simulink model "PID_controler"  (R2022b)
settings: Solver=FixedStepAuto  StartTime=0.0  StopTime=10.0  FixedStep=1e-3  MaxStep=1e-3  RelTol=1e-3
(part 1 of 2)
settings Model: Creator=MAAM  LastModifiedBy=MAAM

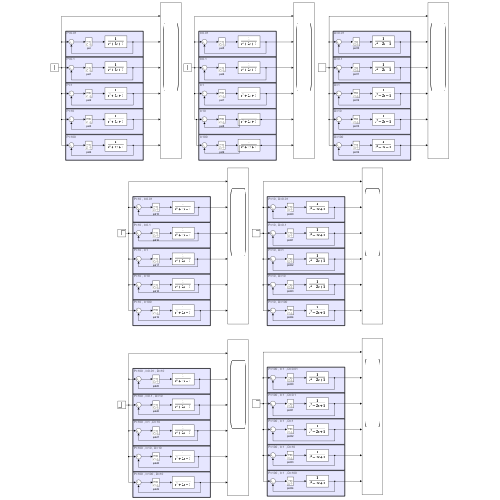
[thumbnail: Simulink's stored preview of the top-level diagram]
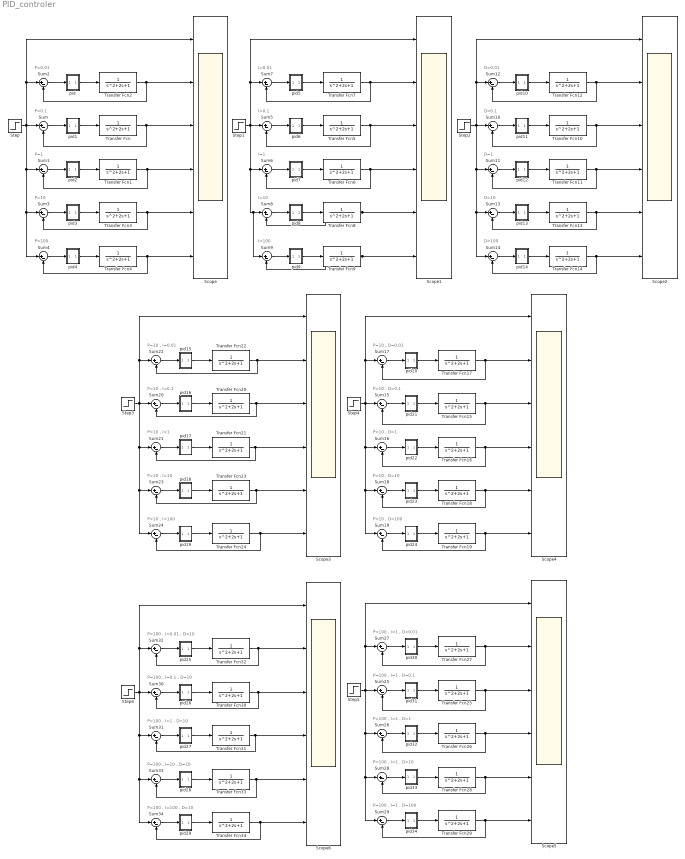
== system PID_controler ==
  note: P=0.1
  note: P=1
  note: P=0.01
  note: P=10
  note: P=100
  note: I=0.1
  note: I=1
  note: I=0.01
  note: I=10
  note: I=100
  note: D=0.1
  note: D=1
  note: D=0.01
  note: D=10
  note: D=100
  note: P=10 , I=0.1
  note: P=10 , I=1
  note: P=10 , I=0.01
  note: P=10 , I=10
  note: P=10 , I=100
  note: P=10 , D=0.1
  note: P=10 , D=1
  note: P=10 , D=0.01
  note: P=10 , D=10
  note: P=10 , D=100
  note: P=100 , I=1 , D=0.1
  note: P=100 , I=1 , D=1
  note: P=100 , I=1 , D=0.01
  note: P=100 , I=1 , D=10
  note: P=100 , I=1 , D=100
  note: P=100 , I=0.1 , D=10
  note: P=100 , I=1 , D=10
  note: P=100 , I=0.01 , D=10
  note: P=100 , I=10 , D=10
  note: P=100 , I=100 , D=10
  Scope{,1..6} (7 alike) : Scope  NumInputPorts=6
  Step{,1..6} (7 alike) : Step  SampleTime=0
  Sum{,1..34} (35 alike) : Sum  Inputs=|+-
  Transfer Fcn{,1..34} (35 alike) : TransferFcn
  pid : Subsystem  Variant=on  mask{F=Parallel, P=0.01, I=0, D=0}
      mask prompts: F "Form"; P "Propotional (P):"; I "Integral      (I):"; D "Drivative    (D):"
      mask init:
      | % Ensure parameters are initialized correctly
      | if isempty(P)
      |     P = 0;
      | end
      | if isempty(I)
      |     I = 0;
      | end
      | if isempty(D)
      |     D = 0;
      | end
      mask TypeOptions F: Parallel | Series | Ideal
      mask TypeOptions P: Subsystem/Gain/Gain | Subsystem1/Gain/Gain | Subsystem2/Gain/Gain
      mask TypeOptions I: Subsystem/Gain1/Gain | Subsystem1/Gain1/Gain | Subsystem2/Gain1/Gain
      mask TypeOptions D: Subsystem/Gain2/Gain | Subsystem1/Gain2/Gain | Subsystem2/Gain2/Gain
      mask Display: fprintf('PID');
  pid1 : Subsystem  Variant=on  mask{F=Parallel, P=0.1, I=0, D=0}
      mask prompts: F "Form"; P "Propotional (P):"; I "Integral      (I):"; D "Drivative    (D):"
      mask init:
      | % Ensure parameters are initialized correctly
      | if isempty(P)
      |     P = 0;
      | end
      | if isempty(I)
      |     I = 0;
      | end
      | if isempty(D)
      |     D = 0;
      | end
      mask TypeOptions F: Parallel | Series | Ideal
      mask TypeOptions P: Subsystem/Gain/Gain | Subsystem1/Gain/Gain | Subsystem2/Gain/Gain
      mask TypeOptions I: Subsystem/Gain1/Gain | Subsystem1/Gain1/Gain | Subsystem2/Gain1/Gain
      mask TypeOptions D: Subsystem/Gain2/Gain | Subsystem1/Gain2/Gain | Subsystem2/Gain2/Gain
      mask Display: fprintf('PID');
  pid10 : Subsystem  Variant=on  mask{F=Parallel, P=0, I=0, D=0.01}
      mask prompts: F "Form"; P "Propotional (P):"; I "Integral      (I):"; D "Drivative    (D):"
      mask init:
      | % Ensure parameters are initialized correctly
      | if isempty(P)
      |     P = 0;
      | end
      | if isempty(I)
      |     I = 0;
      | end
      | if isempty(D)
      |     D = 0;
      | end
      mask TypeOptions F: Parallel | Series | Ideal
      mask TypeOptions P: Subsystem/Gain/Gain | Subsystem1/Gain/Gain | Subsystem2/Gain/Gain
      mask TypeOptions I: Subsystem/Gain1/Gain | Subsystem1/Gain1/Gain | Subsystem2/Gain1/Gain
      mask TypeOptions D: Subsystem/Gain2/Gain | Subsystem1/Gain2/Gain | Subsystem2/Gain2/Gain
      mask Display: fprintf('PID');
  pid11 : Subsystem  Variant=on  mask{F=Parallel, P=0, I=0, D=0.1}
      mask prompts: F "Form"; P "Propotional (P):"; I "Integral      (I):"; D "Drivative    (D):"
      mask init:
      | % Ensure parameters are initialized correctly
      | if isempty(P)
      |     P = 0;
      | end
      | if isempty(I)
      |     I = 0;
      | end
      | if isempty(D)
      |     D = 0;
      | end
      mask TypeOptions F: Parallel | Series | Ideal
      mask TypeOptions P: Subsystem/Gain/Gain | Subsystem1/Gain/Gain | Subsystem2/Gain/Gain
      mask TypeOptions I: Subsystem/Gain1/Gain | Subsystem1/Gain1/Gain | Subsystem2/Gain1/Gain
      mask TypeOptions D: Subsystem/Gain2/Gain | Subsystem1/Gain2/Gain | Subsystem2/Gain2/Gain
      mask Display: fprintf('PID');
  pid12 : Subsystem  Variant=on  mask{F=Parallel, P=0, I=0, D=1}
      mask prompts: F "Form"; P "Propotional (P):"; I "Integral      (I):"; D "Drivative    (D):"
      mask init:
      | % Ensure parameters are initialized correctly
      | if isempty(P)
      |     P = 0;
      | end
      | if isempty(I)
      |     I = 0;
      | end
      | if isempty(D)
      |     D = 0;
      | end
      mask TypeOptions F: Parallel | Series | Ideal
      mask TypeOptions P: Subsystem/Gain/Gain | Subsystem1/Gain/Gain | Subsystem2/Gain/Gain
      mask TypeOptions I: Subsystem/Gain1/Gain | Subsystem1/Gain1/Gain | Subsystem2/Gain1/Gain
      mask TypeOptions D: Subsystem/Gain2/Gain | Subsystem1/Gain2/Gain | Subsystem2/Gain2/Gain
      mask Display: fprintf('PID');
  pid13 : Subsystem  Variant=on  mask{F=Parallel, P=0, I=0, D=10}
      mask prompts: F "Form"; P "Propotional (P):"; I "Integral      (I):"; D "Drivative    (D):"
      mask init:
      | % Ensure parameters are initialized correctly
      | if isempty(P)
      |     P = 0;
      | end
      | if isempty(I)
      |     I = 0;
      | end
      | if isempty(D)
      |     D = 0;
      | end
      mask TypeOptions F: Parallel | Series | Ideal
      mask TypeOptions P: Subsystem/Gain/Gain | Subsystem1/Gain/Gain | Subsystem2/Gain/Gain
      mask TypeOptions I: Subsystem/Gain1/Gain | Subsystem1/Gain1/Gain | Subsystem2/Gain1/Gain
      mask TypeOptions D: Subsystem/Gain2/Gain | Subsystem1/Gain2/Gain | Subsystem2/Gain2/Gain
      mask Display: fprintf('PID');
  pid14 : Subsystem  Variant=on  mask{F=Parallel, P=0, I=0, D=100}
      mask prompts: F "Form"; P "Propotional (P):"; I "Integral      (I):"; D "Drivative    (D):"
      mask init:
      | % Ensure parameters are initialized correctly
      | if isempty(P)
      |     P = 0;
      | end
      | if isempty(I)
      |     I = 0;
      | end
      | if isempty(D)
      |     D = 0;
      | end
      mask TypeOptions F: Parallel | Series | Ideal
      mask TypeOptions P: Subsystem/Gain/Gain | Subsystem1/Gain/Gain | Subsystem2/Gain/Gain
      mask TypeOptions I: Subsystem/Gain1/Gain | Subsystem1/Gain1/Gain | Subsystem2/Gain1/Gain
      mask TypeOptions D: Subsystem/Gain2/Gain | Subsystem1/Gain2/Gain | Subsystem2/Gain2/Gain
      mask Display: fprintf('PID');
  pid15 : Subsystem  Variant=on  mask{F=Parallel, P=100, I=0.01, D=0}
      mask prompts: F "Form"; P "Propotional (P):"; I "Integral      (I):"; D "Drivative    (D):"
      mask init:
      | % Ensure parameters are initialized correctly
      | if isempty(P)
      |     P = 0;
      | end
      | if isempty(I)
      |     I = 0;
      | end
      | if isempty(D)
      |     D = 0;
      | end
      mask TypeOptions F: Parallel | Series | Ideal
      mask TypeOptions P: Subsystem/Gain/Gain | Subsystem1/Gain/Gain | Subsystem2/Gain/Gain
      mask TypeOptions I: Subsystem/Gain1/Gain | Subsystem1/Gain1/Gain | Subsystem2/Gain1/Gain
      mask TypeOptions D: Subsystem/Gain2/Gain | Subsystem1/Gain2/Gain | Subsystem2/Gain2/Gain
      mask Display: fprintf('PID');
  pid16 : Subsystem  Variant=on  mask{F=Parallel, P=100, I=0.1, D=0}
      mask prompts: F "Form"; P "Propotional (P):"; I "Integral      (I):"; D "Drivative    (D):"
      mask init:
      | % Ensure parameters are initialized correctly
      | if isempty(P)
      |     P = 0;
      | end
      | if isempty(I)
      |     I = 0;
      | end
      | if isempty(D)
      |     D = 0;
      | end
      mask TypeOptions F: Parallel | Series | Ideal
      mask TypeOptions P: Subsystem/Gain/Gain | Subsystem1/Gain/Gain | Subsystem2/Gain/Gain
      mask TypeOptions I: Subsystem/Gain1/Gain | Subsystem1/Gain1/Gain | Subsystem2/Gain1/Gain
      mask TypeOptions D: Subsystem/Gain2/Gain | Subsystem1/Gain2/Gain | Subsystem2/Gain2/Gain
      mask Display: fprintf('PID');
  pid17 : Subsystem  Variant=on  mask{F=Parallel, P=100, I=1, D=0}
      mask prompts: F "Form"; P "Propotional (P):"; I "Integral      (I):"; D "Drivative    (D):"
      mask init:
      | % Ensure parameters are initialized correctly
      | if isempty(P)
      |     P = 0;
      | end
      | if isempty(I)
      |     I = 0;
      | end
      | if isempty(D)
      |     D = 0;
      | end
      mask TypeOptions F: Parallel | Series | Ideal
      mask TypeOptions P: Subsystem/Gain/Gain | Subsystem1/Gain/Gain | Subsystem2/Gain/Gain
      mask TypeOptions I: Subsystem/Gain1/Gain | Subsystem1/Gain1/Gain | Subsystem2/Gain1/Gain
      mask TypeOptions D: Subsystem/Gain2/Gain | Subsystem1/Gain2/Gain | Subsystem2/Gain2/Gain
      mask Display: fprintf('PID');
  pid18 : Subsystem  Variant=on  mask{F=Parallel, P=100, I=10, D=0}
      mask prompts: F "Form"; P "Propotional (P):"; I "Integral      (I):"; D "Drivative    (D):"
      mask init:
      | % Ensure parameters are initialized correctly
      | if isempty(P)
      |     P = 0;
      | end
      | if isempty(I)
      |     I = 0;
      | end
      | if isempty(D)
      |     D = 0;
      | end
      mask TypeOptions F: Parallel | Series | Ideal
      mask TypeOptions P: Subsystem/Gain/Gain | Subsystem1/Gain/Gain | Subsystem2/Gain/Gain
      mask TypeOptions I: Subsystem/Gain1/Gain | Subsystem1/Gain1/Gain | Subsystem2/Gain1/Gain
      mask TypeOptions D: Subsystem/Gain2/Gain | Subsystem1/Gain2/Gain | Subsystem2/Gain2/Gain
      mask Display: fprintf('PID');
  pid19 : Subsystem  Variant=on  mask{F=Parallel, P=100, I=100, D=0}
      mask prompts: F "Form"; P "Propotional (P):"; I "Integral      (I):"; D "Drivative    (D):"
      mask init:
      | % Ensure parameters are initialized correctly
      | if isempty(P)
      |     P = 0;
      | end
      | if isempty(I)
      |     I = 0;
      | end
      | if isempty(D)
      |     D = 0;
      | end
      mask TypeOptions F: Parallel | Series | Ideal
      mask TypeOptions P: Subsystem/Gain/Gain | Subsystem1/Gain/Gain | Subsystem2/Gain/Gain
      mask TypeOptions I: Subsystem/Gain1/Gain | Subsystem1/Gain1/Gain | Subsystem2/Gain1/Gain
      mask TypeOptions D: Subsystem/Gain2/Gain | Subsystem1/Gain2/Gain | Subsystem2/Gain2/Gain
      mask Display: fprintf('PID');
  pid2 : Subsystem  Variant=on  mask{F=Parallel, P=1, I=0, D=0}
      mask prompts: F "Form"; P "Propotional (P):"; I "Integral      (I):"; D "Drivative    (D):"
      mask init:
      | % Ensure parameters are initialized correctly
      | if isempty(P)
      |     P = 0;
      | end
      | if isempty(I)
      |     I = 0;
      | end
      | if isempty(D)
      |     D = 0;
      | end
      mask TypeOptions F: Parallel | Series | Ideal
      mask TypeOptions P: Subsystem/Gain/Gain | Subsystem1/Gain/Gain | Subsystem2/Gain/Gain
      mask TypeOptions I: Subsystem/Gain1/Gain | Subsystem1/Gain1/Gain | Subsystem2/Gain1/Gain
      mask TypeOptions D: Subsystem/Gain2/Gain | Subsystem1/Gain2/Gain | Subsystem2/Gain2/Gain
      mask Display: fprintf('PID');
  pid20 : Subsystem  Variant=on  mask{F=Parallel, P=100, I=0, D=0.01}
      mask prompts: F "Form"; P "Propotional (P):"; I "Integral      (I):"; D "Drivative    (D):"
      mask init:
      | % Ensure parameters are initialized correctly
      | if isempty(P)
      |     P = 0;
      | end
      | if isempty(I)
      |     I = 0;
      | end
      | if isempty(D)
      |     D = 0;
      | end
      mask TypeOptions F: Parallel | Series | Ideal
      mask TypeOptions P: Subsystem/Gain/Gain | Subsystem1/Gain/Gain | Subsystem2/Gain/Gain
      mask TypeOptions I: Subsystem/Gain1/Gain | Subsystem1/Gain1/Gain | Subsystem2/Gain1/Gain
      mask TypeOptions D: Subsystem/Gain2/Gain | Subsystem1/Gain2/Gain | Subsystem2/Gain2/Gain
      mask Display: fprintf('PID');
  pid21 : Subsystem  Variant=on  mask{F=Parallel, P=100, I=0, D=0.1}
      mask prompts: F "Form"; P "Propotional (P):"; I "Integral      (I):"; D "Drivative    (D):"
      mask init:
      | % Ensure parameters are initialized correctly
      | if isempty(P)
      |     P = 0;
      | end
      | if isempty(I)
      |     I = 0;
      | end
      | if isempty(D)
      |     D = 0;
      | end
      mask TypeOptions F: Parallel | Series | Ideal
      mask TypeOptions P: Subsystem/Gain/Gain | Subsystem1/Gain/Gain | Subsystem2/Gain/Gain
      mask TypeOptions I: Subsystem/Gain1/Gain | Subsystem1/Gain1/Gain | Subsystem2/Gain1/Gain
      mask TypeOptions D: Subsystem/Gain2/Gain | Subsystem1/Gain2/Gain | Subsystem2/Gain2/Gain
      mask Display: fprintf('PID');
  pid22 : Subsystem  Variant=on  mask{F=Parallel, P=100, I=0, D=1}
      mask prompts: F "Form"; P "Propotional (P):"; I "Integral      (I):"; D "Drivative    (D):"
      mask init:
      | % Ensure parameters are initialized correctly
      | if isempty(P)
      |     P = 0;
      | end
      | if isempty(I)
      |     I = 0;
      | end
      | if isempty(D)
      |     D = 0;
      | end
      mask TypeOptions F: Parallel | Series | Ideal
      mask TypeOptions P: Subsystem/Gain/Gain | Subsystem1/Gain/Gain | Subsystem2/Gain/Gain
      mask TypeOptions I: Subsystem/Gain1/Gain | Subsystem1/Gain1/Gain | Subsystem2/Gain1/Gain
      mask TypeOptions D: Subsystem/Gain2/Gain | Subsystem1/Gain2/Gain | Subsystem2/Gain2/Gain
      mask Display: fprintf('PID');
  pid23 : Subsystem  Variant=on  mask{F=Parallel, P=100, I=0, D=10}
      mask prompts: F "Form"; P "Propotional (P):"; I "Integral      (I):"; D "Drivative    (D):"
      mask init:
      | % Ensure parameters are initialized correctly
      | if isempty(P)
      |     P = 0;
      | end
      | if isempty(I)
      |     I = 0;
      | end
      | if isempty(D)
      |     D = 0;
      | end
      mask TypeOptions F: Parallel | Series | Ideal
      mask TypeOptions P: Subsystem/Gain/Gain | Subsystem1/Gain/Gain | Subsystem2/Gain/Gain
      mask TypeOptions I: Subsystem/Gain1/Gain | Subsystem1/Gain1/Gain | Subsystem2/Gain1/Gain
      mask TypeOptions D: Subsystem/Gain2/Gain | Subsystem1/Gain2/Gain | Subsystem2/Gain2/Gain
      mask Display: fprintf('PID');
  pid24 : Subsystem  Variant=on  mask{F=Parallel, P=100, I=0, D=100}
      mask prompts: F "Form"; P "Propotional (P):"; I "Integral      (I):"; D "Drivative    (D):"
      mask init:
      | % Ensure parameters are initialized correctly
      | if isempty(P)
      |     P = 0;
      | end
      | if isempty(I)
      |     I = 0;
      | end
      | if isempty(D)
      |     D = 0;
      | end
      mask TypeOptions F: Parallel | Series | Ideal
      mask TypeOptions P: Subsystem/Gain/Gain | Subsystem1/Gain/Gain | Subsystem2/Gain/Gain
      mask TypeOptions I: Subsystem/Gain1/Gain | Subsystem1/Gain1/Gain | Subsystem2/Gain1/Gain
      mask TypeOptions D: Subsystem/Gain2/Gain | Subsystem1/Gain2/Gain | Subsystem2/Gain2/Gain
      mask Display: fprintf('PID');
  pid25 : Subsystem  Variant=on  mask{F=Parallel, P=100, I=0.01, D=10}
      mask prompts: F "Form"; P "Propotional (P):"; I "Integral      (I):"; D "Drivative    (D):"
      mask init:
      | % Ensure parameters are initialized correctly
      | if isempty(P)
      |     P = 0;
      | end
      | if isempty(I)
      |     I = 0;
      | end
      | if isempty(D)
      |     D = 0;
      | end
      mask TypeOptions F: Parallel | Series | Ideal
      mask TypeOptions P: Subsystem/Gain/Gain | Subsystem1/Gain/Gain | Subsystem2/Gain/Gain
      mask TypeOptions I: Subsystem/Gain1/Gain | Subsystem1/Gain1/Gain | Subsystem2/Gain1/Gain
      mask TypeOptions D: Subsystem/Gain2/Gain | Subsystem1/Gain2/Gain | Subsystem2/Gain2/Gain
      mask Display: fprintf('PID');
  pid26 : Subsystem  Variant=on  mask{F=Parallel, P=100, I=0.1, D=10}
      mask prompts: F "Form"; P "Propotional (P):"; I "Integral      (I):"; D "Drivative    (D):"
      mask init:
      | % Ensure parameters are initialized correctly
      | if isempty(P)
      |     P = 0;
      | end
      | if isempty(I)
      |     I = 0;
      | end
      | if isempty(D)
      |     D = 0;
      | end
      mask TypeOptions F: Parallel | Series | Ideal
      mask TypeOptions P: Subsystem/Gain/Gain | Subsystem1/Gain/Gain | Subsystem2/Gain/Gain
      mask TypeOptions I: Subsystem/Gain1/Gain | Subsystem1/Gain1/Gain | Subsystem2/Gain1/Gain
      mask TypeOptions D: Subsystem/Gain2/Gain | Subsystem1/Gain2/Gain | Subsystem2/Gain2/Gain
      mask Display: fprintf('PID');
  pid27 : Subsystem  Variant=on  mask{F=Parallel, P=100, I=1, D=10}
      mask prompts: F "Form"; P "Propotional (P):"; I "Integral      (I):"; D "Drivative    (D):"
      mask init:
      | % Ensure parameters are initialized correctly
      | if isempty(P)
      |     P = 0;
      | end
      | if isempty(I)
      |     I = 0;
      | end
      | if isempty(D)
      |     D = 0;
      | end
      mask TypeOptions F: Parallel | Series | Ideal
      mask TypeOptions P: Subsystem/Gain/Gain | Subsystem1/Gain/Gain | Subsystem2/Gain/Gain
      mask TypeOptions I: Subsystem/Gain1/Gain | Subsystem1/Gain1/Gain | Subsystem2/Gain1/Gain
      mask TypeOptions D: Subsystem/Gain2/Gain | Subsystem1/Gain2/Gain | Subsystem2/Gain2/Gain
      mask Display: fprintf('PID');
  pid28 : Subsystem  Variant=on  mask{F=Parallel, P=100, I=10, D=10}
      mask prompts: F "Form"; P "Propotional (P):"; I "Integral      (I):"; D "Drivative    (D):"
      mask init:
      | % Ensure parameters are initialized correctly
      | if isempty(P)
      |     P = 0;
      | end
      | if isempty(I)
      |     I = 0;
      | end
      | if isempty(D)
      |     D = 0;
      | end
      mask TypeOptions F: Parallel | Series | Ideal
      mask TypeOptions P: Subsystem/Gain/Gain | Subsystem1/Gain/Gain | Subsystem2/Gain/Gain
      mask TypeOptions I: Subsystem/Gain1/Gain | Subsystem1/Gain1/Gain | Subsystem2/Gain1/Gain
      mask TypeOptions D: Subsystem/Gain2/Gain | Subsystem1/Gain2/Gain | Subsystem2/Gain2/Gain
      mask Display: fprintf('PID');
  pid29 : Subsystem  Variant=on  mask{F=Parallel, P=100, I=100, D=10}
      mask prompts: F "Form"; P "Propotional (P):"; I "Integral      (I):"; D "Drivative    (D):"
      mask init:
      | % Ensure parameters are initialized correctly
      | if isempty(P)
      |     P = 0;
      | end
      | if isempty(I)
      |     I = 0;
      | end
      | if isempty(D)
      |     D = 0;
      | end
      mask TypeOptions F: Parallel | Series | Ideal
      mask TypeOptions P: Subsystem/Gain/Gain | Subsystem1/Gain/Gain | Subsystem2/Gain/Gain
      mask TypeOptions I: Subsystem/Gain1/Gain | Subsystem1/Gain1/Gain | Subsystem2/Gain1/Gain
      mask TypeOptions D: Subsystem/Gain2/Gain | Subsystem1/Gain2/Gain | Subsystem2/Gain2/Gain
      mask Display: fprintf('PID');
  pid3 : Subsystem  Variant=on  mask{F=Parallel, P=10, I=0, D=0}
      mask prompts: F "Form"; P "Propotional (P):"; I "Integral      (I):"; D "Drivative    (D):"
      mask init:
      | % Ensure parameters are initialized correctly
      | if isempty(P)
      |     P = 0;
      | end
      | if isempty(I)
      |     I = 0;
      | end
      | if isempty(D)
      |     D = 0;
      | end
      mask TypeOptions F: Parallel | Series | Ideal
      mask TypeOptions P: Subsystem/Gain/Gain | Subsystem1/Gain/Gain | Subsystem2/Gain/Gain
      mask TypeOptions I: Subsystem/Gain1/Gain | Subsystem1/Gain1/Gain | Subsystem2/Gain1/Gain
      mask TypeOptions D: Subsystem/Gain2/Gain | Subsystem1/Gain2/Gain | Subsystem2/Gain2/Gain
      mask Display: fprintf('PID');
  pid30 : Subsystem  Variant=on  mask{F=Parallel, P=100, I=1, D=0.01}
      mask prompts: F "Form"; P "Propotional (P):"; I "Integral      (I):"; D "Drivative    (D):"
      mask init:
      | % Ensure parameters are initialized correctly
      | if isempty(P)
      |     P = 0;
      | end
      | if isempty(I)
      |     I = 0;
      | end
      | if isempty(D)
      |     D = 0;
      | end
      mask TypeOptions F: Parallel | Series | Ideal
      mask TypeOptions P: Subsystem/Gain/Gain | Subsystem1/Gain/Gain | Subsystem2/Gain/Gain
      mask TypeOptions I: Subsystem/Gain1/Gain | Subsystem1/Gain1/Gain | Subsystem2/Gain1/Gain
      mask TypeOptions D: Subsystem/Gain2/Gain | Subsystem1/Gain2/Gain | Subsystem2/Gain2/Gain
      mask Display: fprintf('PID');
  pid31 : Subsystem  Variant=on  mask{F=Parallel, P=100, I=1, D=0.1}
      mask prompts: F "Form"; P "Propotional (P):"; I "Integral      (I):"; D "Drivative    (D):"
      mask init:
      | % Ensure parameters are initialized correctly
      | if isempty(P)
      |     P = 0;
      | end
      | if isempty(I)
      |     I = 0;
      | end
      | if isempty(D)
      |     D = 0;
      | end
      mask TypeOptions F: Parallel | Series | Ideal
      mask TypeOptions P: Subsystem/Gain/Gain | Subsystem1/Gain/Gain | Subsystem2/Gain/Gain
      mask TypeOptions I: Subsystem/Gain1/Gain | Subsystem1/Gain1/Gain | Subsystem2/Gain1/Gain
      mask TypeOptions D: Subsystem/Gain2/Gain | Subsystem1/Gain2/Gain | Subsystem2/Gain2/Gain
      mask Display: fprintf('PID');
  pid32 : Subsystem  Variant=on  mask{F=Parallel, P=100, I=1, D=1}
      mask prompts: F "Form"; P "Propotional (P):"; I "Integral      (I):"; D "Drivative    (D):"
      mask init:
      | % Ensure parameters are initialized correctly
      | if isempty(P)
      |     P = 0;
      | end
      | if isempty(I)
      |     I = 0;
      | end
      | if isempty(D)
      |     D = 0;
      | end
      mask TypeOptions F: Parallel | Series | Ideal
      mask TypeOptions P: Subsystem/Gain/Gain | Subsystem1/Gain/Gain | Subsystem2/Gain/Gain
      mask TypeOptions I: Subsystem/Gain1/Gain | Subsystem1/Gain1/Gain | Subsystem2/Gain1/Gain
      mask TypeOptions D: Subsystem/Gain2/Gain | Subsystem1/Gain2/Gain | Subsystem2/Gain2/Gain
      mask Display: fprintf('PID');
  pid33 : Subsystem  Variant=on  mask{F=Parallel, P=100, I=1, D=10}
      mask prompts: F "Form"; P "Propotional (P):"; I "Integral      (I):"; D "Drivative    (D):"
      mask init:
      | % Ensure parameters are initialized correctly
      | if isempty(P)
      |     P = 0;
      | end
      | if isempty(I)
      |     I = 0;
      | end
      | if isempty(D)
      |     D = 0;
      | end
      mask TypeOptions F: Parallel | Series | Ideal
      mask TypeOptions P: Subsystem/Gain/Gain | Subsystem1/Gain/Gain | Subsystem2/Gain/Gain
      mask TypeOptions I: Subsystem/Gain1/Gain | Subsystem1/Gain1/Gain | Subsystem2/Gain1/Gain
      mask TypeOptions D: Subsystem/Gain2/Gain | Subsystem1/Gain2/Gain | Subsystem2/Gain2/Gain
      mask Display: fprintf('PID');
  pid34 : Subsystem  Variant=on  mask{F=Parallel, P=100, I=1, D=100}
      mask prompts: F "Form"; P "Propotional (P):"; I "Integral      (I):"; D "Drivative    (D):"
      mask init:
      | % Ensure parameters are initialized correctly
      | if isempty(P)
      |     P = 0;
      | end
      | if isempty(I)
      |     I = 0;
      | end
      | if isempty(D)
      |     D = 0;
      | end
      mask TypeOptions F: Parallel | Series | Ideal
      mask TypeOptions P: Subsystem/Gain/Gain | Subsystem1/Gain/Gain | Subsystem2/Gain/Gain
      mask TypeOptions I: Subsystem/Gain1/Gain | Subsystem1/Gain1/Gain | Subsystem2/Gain1/Gain
      mask TypeOptions D: Subsystem/Gain2/Gain | Subsystem1/Gain2/Gain | Subsystem2/Gain2/Gain
      mask Display: fprintf('PID');
  pid4 : Subsystem  Variant=on  mask{F=Parallel, P=100, I=0, D=0}
      mask prompts: F "Form"; P "Propotional (P):"; I "Integral      (I):"; D "Drivative    (D):"
      mask init:
      | % Ensure parameters are initialized correctly
      | if isempty(P)
      |     P = 0;
      | end
      | if isempty(I)
      |     I = 0;
      | end
      | if isempty(D)
      |     D = 0;
      | end
      mask TypeOptions F: Parallel | Series | Ideal
      mask TypeOptions P: Subsystem/Gain/Gain | Subsystem1/Gain/Gain | Subsystem2/Gain/Gain
      mask TypeOptions I: Subsystem/Gain1/Gain | Subsystem1/Gain1/Gain | Subsystem2/Gain1/Gain
      mask TypeOptions D: Subsystem/Gain2/Gain | Subsystem1/Gain2/Gain | Subsystem2/Gain2/Gain
      mask Display: fprintf('PID');
  pid5 : Subsystem  Variant=on  mask{F=Parallel, P=0, I=0.01, D=0}
      mask prompts: F "Form"; P "Propotional (P):"; I "Integral      (I):"; D "Drivative    (D):"
      mask init:
      | % Ensure parameters are initialized correctly
      | if isempty(P)
      |     P = 0;
      | end
      | if isempty(I)
      |     I = 0;
      | end
      | if isempty(D)
      |     D = 0;
      | end
      mask TypeOptions F: Parallel | Series | Ideal
      mask TypeOptions P: Subsystem/Gain/Gain | Subsystem1/Gain/Gain | Subsystem2/Gain/Gain
      mask TypeOptions I: Subsystem/Gain1/Gain | Subsystem1/Gain1/Gain | Subsystem2/Gain1/Gain
      mask TypeOptions D: Subsystem/Gain2/Gain | Subsystem1/Gain2/Gain | Subsystem2/Gain2/Gain
      mask Display: fprintf('PID');
  pid6 : Subsystem  Variant=on  mask{F=Parallel, P=0, I=0.1, D=0}
      mask prompts: F "Form"; P "Propotional (P):"; I "Integral      (I):"; D "Drivative    (D):"
      mask init:
      | % Ensure parameters are initialized correctly
      | if isempty(P)
      |     P = 0;
      | end
      | if isempty(I)
      |     I = 0;
      | end
      | if isempty(D)
      |     D = 0;
      | end
      mask TypeOptions F: Parallel | Series | Ideal
      mask TypeOptions P: Subsystem/Gain/Gain | Subsystem1/Gain/Gain | Subsystem2/Gain/Gain
      mask TypeOptions I: Subsystem/Gain1/Gain | Subsystem1/Gain1/Gain | Subsystem2/Gain1/Gain
      mask TypeOptions D: Subsystem/Gain2/Gain | Subsystem1/Gain2/Gain | Subsystem2/Gain2/Gain
      mask Display: fprintf('PID');
  pid7 : Subsystem  Variant=on  mask{F=Parallel, P=0, I=1, D=0}
      mask prompts: F "Form"; P "Propotional (P):"; I "Integral      (I):"; D "Drivative    (D):"
      mask init:
      | % Ensure parameters are initialized correctly
      | if isempty(P)
      |     P = 0;
      | end
      | if isempty(I)
      |     I = 0;
      | end
      | if isempty(D)
      |     D = 0;
      | end
      mask TypeOptions F: Parallel | Series | Ideal
      mask TypeOptions P: Subsystem/Gain/Gain | Subsystem1/Gain/Gain | Subsystem2/Gain/Gain
      mask TypeOptions I: Subsystem/Gain1/Gain | Subsystem1/Gain1/Gain | Subsystem2/Gain1/Gain
      mask TypeOptions D: Subsystem/Gain2/Gain | Subsystem1/Gain2/Gain | Subsystem2/Gain2/Gain
      mask Display: fprintf('PID');
  pid8 : Subsystem  Variant=on  mask{F=Parallel, P=0, I=10, D=0}
      mask prompts: F "Form"; P "Propotional (P):"; I "Integral      (I):"; D "Drivative    (D):"
      mask init:
      | % Ensure parameters are initialized correctly
      | if isempty(P)
      |     P = 0;
      | end
      | if isempty(I)
      |     I = 0;
      | end
      | if isempty(D)
      |     D = 0;
      | end
      mask TypeOptions F: Parallel | Series | Ideal
      mask TypeOptions P: Subsystem/Gain/Gain | Subsystem1/Gain/Gain | Subsystem2/Gain/Gain
      mask TypeOptions I: Subsystem/Gain1/Gain | Subsystem1/Gain1/Gain | Subsystem2/Gain1/Gain
      mask TypeOptions D: Subsystem/Gain2/Gain | Subsystem1/Gain2/Gain | Subsystem2/Gain2/Gain
      mask Display: fprintf('PID');
  pid9 : Subsystem  Variant=on  mask{F=Parallel, P=0, I=0, D=100}
      mask prompts: F "Form"; P "Propotional (P):"; I "Integral      (I):"; D "Drivative    (D):"
      mask init:
      | % Ensure parameters are initialized correctly
      | if isempty(P)
      |     P = 0;
      | end
      | if isempty(I)
      |     I = 0;
      | end
      | if isempty(D)
      |     D = 0;
      | end
      mask TypeOptions F: Parallel | Series | Ideal
      mask TypeOptions P: Subsystem/Gain/Gain | Subsystem1/Gain/Gain | Subsystem2/Gain/Gain
      mask TypeOptions I: Subsystem/Gain1/Gain | Subsystem1/Gain1/Gain | Subsystem2/Gain1/Gain
      mask TypeOptions D: Subsystem/Gain2/Gain | Subsystem1/Gain2/Gain | Subsystem2/Gain2/Gain
      mask Display: fprintf('PID');
  wires:
  Step/1 -> Sum3/1, Sum4/1, Sum1/1, Sum2/1, Scope/1, Sum/1
  Transfer Fcn/1 -> Sum/2, Scope/3
  Sum/1 -> pid1/1(In1)
  pid1/1(Out1) -> Transfer Fcn/1
  pid2/1(Out1) -> Transfer Fcn1/1
  Sum1/1 -> pid2/1(In1)
  pid/1(Out1) -> Transfer Fcn2/1
  Sum2/1 -> pid/1(In1)
  Transfer Fcn2/1 -> Sum2/2, Scope/2
  Transfer Fcn1/1 -> Sum1/2, Scope/4
  Sum3/1 -> pid3/1(In1)
  pid3/1(Out1) -> Transfer Fcn3/1
  pid4/1(Out1) -> Transfer Fcn4/1
  Sum4/1 -> pid4/1(In1)
  Transfer Fcn3/1 -> Sum3/2, Scope/5
  Transfer Fcn4/1 -> Sum4/2, Scope/6
  Transfer Fcn9/1 -> Scope1/6, Sum9/2
  Transfer Fcn8/1 -> Scope1/5, Sum8/2
  Sum9/1 -> pid9/1(In1)
  pid9/1(Out1) -> Transfer Fcn9/1
  pid8/1(Out1) -> Transfer Fcn8/1
  Sum8/1 -> pid8/1(In1)
  Transfer Fcn6/1 -> Scope1/4, Sum6/2
  Transfer Fcn7/1 -> Scope1/2, Sum7/2
  Sum7/1 -> pid5/1(In1)
  pid5/1(Out1) -> Transfer Fcn7/1
  Sum6/1 -> pid7/1(In1)
  pid7/1(Out1) -> Transfer Fcn6/1
  pid6/1(Out1) -> Transfer Fcn5/1
  Sum5/1 -> pid6/1(In1)
  Transfer Fcn5/1 -> Scope1/3, Sum5/2
  Step1/1 -> Sum5/1, Scope1/1, Sum7/1, Sum6/1, Sum9/1, Sum8/1
  Step2/1 -> Sum13/1, Sum14/1, Sum11/1, Sum12/1, Scope2/1, Sum10/1
  Transfer Fcn10/1 -> Sum10/2, Scope2/3
  Sum10/1 -> pid11/1(In1)
  pid11/1(Out1) -> Transfer Fcn10/1
  pid12/1(Out1) -> Transfer Fcn11/1
  Sum11/1 -> pid12/1(In1)
  pid10/1(Out1) -> Transfer Fcn12/1
  Sum12/1 -> pid10/1(In1)
  Transfer Fcn12/1 -> Sum12/2, Scope2/2
  Transfer Fcn11/1 -> Sum11/2, Scope2/4
  Sum13/1 -> pid13/1(In1)
  pid13/1(Out1) -> Transfer Fcn13/1
  pid14/1(Out1) -> Transfer Fcn14/1
  Sum14/1 -> pid14/1(In1)
  Transfer Fcn13/1 -> Sum13/2, Scope2/5
  Transfer Fcn14/1 -> Sum14/2, Scope2/6
  Transfer Fcn19/1 -> Scope4/6, Sum19/2
  Transfer Fcn18/1 -> Scope4/5, Sum18/2
  Sum19/1 -> pid24/1(In1)
  pid24/1(Out1) -> Transfer Fcn19/1
  pid23/1(Out1) -> Transfer Fcn18/1
  Sum18/1 -> pid23/1(In1)
  Transfer Fcn16/1 -> Scope4/4, Sum16/2
  Transfer Fcn17/1 -> Scope4/2, Sum17/2
  Sum17/1 -> pid20/1(In1)
  pid20/1(Out1) -> Transfer Fcn17/1
  Sum16/1 -> pid22/1(In1)
  pid22/1(Out1) -> Transfer Fcn16/1
  pid21/1(Out1) -> Transfer Fcn15/1
  Sum15/1 -> pid21/1(In1)
  Transfer Fcn15/1 -> Scope4/3, Sum15/2
  Step4/1 -> Sum18/1, Sum19/1, Sum16/1, Sum15/1, Sum17/1, Scope4/1
  Step3/1 -> Sum23/1, Sum24/1, Sum21/1, Sum22/1, Scope3/1, Sum20/1
  Transfer Fcn20/1 -> Scope3/3, Sum20/2
  Sum20/1 -> pid16/1(In1)
  pid16/1(Out1) -> Transfer Fcn20/1
  pid17/1(Out1) -> Transfer Fcn21/1
  Sum21/1 -> pid17/1(In1)
  pid15/1(Out1) -> Transfer Fcn22/1
  Sum22/1 -> pid15/1(In1)
  Transfer Fcn22/1 -> Scope3/2, Sum22/2
  Transfer Fcn21/1 -> Scope3/4, Sum21/2
  Sum23/1 -> pid18/1(In1)
  pid18/1(Out1) -> Transfer Fcn23/1
  pid19/1(Out1) -> Transfer Fcn24/1
  Sum24/1 -> pid19/1(In1)
  Transfer Fcn23/1 -> Scope3/5, Sum23/2
  Transfer Fcn24/1 -> Sum24/2, Scope3/6
  Step5/1 -> Sum28/1, Sum29/1, Sum26/1, Sum27/1, Scope5/1, Sum25/1
  Transfer Fcn25/1 -> Sum25/2, Scope5/3
  Sum25/1 -> pid31/1(In1)
  pid31/1(Out1) -> Transfer Fcn25/1
  pid32/1(Out1) -> Transfer Fcn26/1
  Sum26/1 -> pid32/1(In1)
  pid30/1(Out1) -> Transfer Fcn27/1
  Sum27/1 -> pid30/1(In1)
  Transfer Fcn27/1 -> Sum27/2, Scope5/2
  Transfer Fcn26/1 -> Sum26/2, Scope5/4
  Sum28/1 -> pid33/1(In1)
  pid33/1(Out1) -> Transfer Fcn28/1
  pid34/1(Out1) -> Transfer Fcn29/1
  Sum29/1 -> pid34/1(In1)
  Transfer Fcn28/1 -> Sum28/2, Scope5/5
  Transfer Fcn29/1 -> Sum29/2, Scope5/6
  Transfer Fcn34/1 -> Scope6/6, Sum34/2
  Transfer Fcn33/1 -> Sum33/2, Scope6/5
  Sum34/1 -> pid29/1(In1)
  pid29/1(Out1) -> Transfer Fcn34/1
  pid28/1(Out1) -> Transfer Fcn33/1
  Sum33/1 -> pid28/1(In1)
  Transfer Fcn31/1 -> Sum31/2, Scope6/4
  Transfer Fcn32/1 -> Sum32/2, Scope6/2
  Sum32/1 -> pid25/1(In1)
  pid25/1(Out1) -> Transfer Fcn32/1
  Sum31/1 -> pid27/1(In1)
  pid27/1(Out1) -> Transfer Fcn31/1
  pid26/1(Out1) -> Transfer Fcn30/1
  Sum30/1 -> pid26/1(In1)
  Transfer Fcn30/1 -> Sum30/2, Scope6/3
  Step6/1 -> Sum30/1, Scope6/1, Sum32/1, Sum31/1, Sum34/1, Sum33/1

== system PID_controler/pid ==
  In1 : Inport
  Subsystem : Subsystem  VariantControl=F==1
  Subsystem1 : Subsystem  VariantControl=F==2
  Subsystem2 : Subsystem  VariantControl=F==3
  Out1 : Outport

== system PID_controler/pid1 ==
  In1 : Inport
  Subsystem : Subsystem  VariantControl=F==1
  Subsystem1 : Subsystem  VariantControl=F==2
  Subsystem2 : Subsystem  VariantControl=F==3
  Out1 : Outport

== system PID_controler/pid10 ==
  In1 : Inport
  Subsystem : Subsystem  VariantControl=F==1
  Subsystem1 : Subsystem  VariantControl=F==2
  Subsystem2 : Subsystem  VariantControl=F==3
  Out1 : Outport

== system PID_controler/pid11 ==
  In1 : Inport
  Subsystem : Subsystem  VariantControl=F==1
  Subsystem1 : Subsystem  VariantControl=F==2
  Subsystem2 : Subsystem  VariantControl=F==3
  Out1 : Outport

== system PID_controler/pid12 ==
  In1 : Inport
  Subsystem : Subsystem  VariantControl=F==1
  Subsystem1 : Subsystem  VariantControl=F==2
  Subsystem2 : Subsystem  VariantControl=F==3
  Out1 : Outport

== system PID_controler/pid13 ==
  In1 : Inport
  Subsystem : Subsystem  VariantControl=F==1
  Subsystem1 : Subsystem  VariantControl=F==2
  Subsystem2 : Subsystem  VariantControl=F==3
  Out1 : Outport

== system PID_controler/pid14 ==
  In1 : Inport
  Subsystem : Subsystem  VariantControl=F==1
  Subsystem1 : Subsystem  VariantControl=F==2
  Subsystem2 : Subsystem  VariantControl=F==3
  Out1 : Outport

== system PID_controler/pid15 ==
  In1 : Inport
  Subsystem : Subsystem  VariantControl=F==1
  Subsystem1 : Subsystem  VariantControl=F==2
  Subsystem2 : Subsystem  VariantControl=F==3
  Out1 : Outport

== system PID_controler/pid16 ==
  In1 : Inport
  Subsystem : Subsystem  VariantControl=F==1
  Subsystem1 : Subsystem  VariantControl=F==2
  Subsystem2 : Subsystem  VariantControl=F==3
  Out1 : Outport

== system PID_controler/pid17 ==
  In1 : Inport
  Subsystem : Subsystem  VariantControl=F==1
  Subsystem1 : Subsystem  VariantControl=F==2
  Subsystem2 : Subsystem  VariantControl=F==3
  Out1 : Outport

== system PID_controler/pid18 ==
  In1 : Inport
  Subsystem : Subsystem  VariantControl=F==1
  Subsystem1 : Subsystem  VariantControl=F==2
  Subsystem2 : Subsystem  VariantControl=F==3
  Out1 : Outport

== system PID_controler/pid19 ==
  In1 : Inport
  Subsystem : Subsystem  VariantControl=F==1
  Subsystem1 : Subsystem  VariantControl=F==2
  Subsystem2 : Subsystem  VariantControl=F==3
  Out1 : Outport

== system PID_controler/pid2 ==
  In1 : Inport
  Subsystem : Subsystem  VariantControl=F==1
  Subsystem1 : Subsystem  VariantControl=F==2
  Subsystem2 : Subsystem  VariantControl=F==3
  Out1 : Outport

== system PID_controler/pid20 ==
  In1 : Inport
  Subsystem : Subsystem  VariantControl=F==1
  Subsystem1 : Subsystem  VariantControl=F==2
  Subsystem2 : Subsystem  VariantControl=F==3
  Out1 : Outport

== system PID_controler/pid21 ==
  In1 : Inport
  Subsystem : Subsystem  VariantControl=F==1
  Subsystem1 : Subsystem  VariantControl=F==2
  Subsystem2 : Subsystem  VariantControl=F==3
  Out1 : Outport

== system PID_controler/pid22 ==
  In1 : Inport
  Subsystem : Subsystem  VariantControl=F==1
  Subsystem1 : Subsystem  VariantControl=F==2
  Subsystem2 : Subsystem  VariantControl=F==3
  Out1 : Outport

== system PID_controler/pid23 ==
  In1 : Inport
  Subsystem : Subsystem  VariantControl=F==1
  Subsystem1 : Subsystem  VariantControl=F==2
  Subsystem2 : Subsystem  VariantControl=F==3
  Out1 : Outport

== system PID_controler/pid24 ==
  In1 : Inport
  Subsystem : Subsystem  VariantControl=F==1
  Subsystem1 : Subsystem  VariantControl=F==2
  Subsystem2 : Subsystem  VariantControl=F==3
  Out1 : Outport

== system PID_controler/pid25 ==
  In1 : Inport
  Subsystem : Subsystem  VariantControl=F==1
  Subsystem1 : Subsystem  VariantControl=F==2
  Subsystem2 : Subsystem  VariantControl=F==3
  Out1 : Outport

== system PID_controler/pid26 ==
  In1 : Inport
  Subsystem : Subsystem  VariantControl=F==1
  Subsystem1 : Subsystem  VariantControl=F==2
  Subsystem2 : Subsystem  VariantControl=F==3
  Out1 : Outport

== system PID_controler/pid27 ==
  In1 : Inport
  Subsystem : Subsystem  VariantControl=F==1
  Subsystem1 : Subsystem  VariantControl=F==2
  Subsystem2 : Subsystem  VariantControl=F==3
  Out1 : Outport

== system PID_controler/pid28 ==
  In1 : Inport
  Subsystem : Subsystem  VariantControl=F==1
  Subsystem1 : Subsystem  VariantControl=F==2
  Subsystem2 : Subsystem  VariantControl=F==3
  Out1 : Outport

== system PID_controler/pid29 ==
  In1 : Inport
  Subsystem : Subsystem  VariantControl=F==1
  Subsystem1 : Subsystem  VariantControl=F==2
  Subsystem2 : Subsystem  VariantControl=F==3
  Out1 : Outport

== system PID_controler/pid3 ==
  In1 : Inport
  Subsystem : Subsystem  VariantControl=F==1
  Subsystem1 : Subsystem  VariantControl=F==2
  Subsystem2 : Subsystem  VariantControl=F==3
  Out1 : Outport

== system PID_controler/pid30 ==
  In1 : Inport
  Subsystem : Subsystem  VariantControl=F==1
  Subsystem1 : Subsystem  VariantControl=F==2
  Subsystem2 : Subsystem  VariantControl=F==3
  Out1 : Outport

== system PID_controler/pid31 ==
  In1 : Inport
  Subsystem : Subsystem  VariantControl=F==1
  Subsystem1 : Subsystem  VariantControl=F==2
  Subsystem2 : Subsystem  VariantControl=F==3
  Out1 : Outport

== system PID_controler/pid32 ==
  In1 : Inport
  Subsystem : Subsystem  VariantControl=F==1
  Subsystem1 : Subsystem  VariantControl=F==2
  Subsystem2 : Subsystem  VariantControl=F==3
  Out1 : Outport

== system PID_controler/pid33 ==
  In1 : Inport
  Subsystem : Subsystem  VariantControl=F==1
  Subsystem1 : Subsystem  VariantControl=F==2
  Subsystem2 : Subsystem  VariantControl=F==3
  Out1 : Outport

== system PID_controler/pid34 ==
  In1 : Inport
  Subsystem : Subsystem  VariantControl=F==1
  Subsystem1 : Subsystem  VariantControl=F==2
  Subsystem2 : Subsystem  VariantControl=F==3
  Out1 : Outport

== system PID_controler/pid4 ==
  In1 : Inport
  Subsystem : Subsystem  VariantControl=F==1
  Subsystem1 : Subsystem  VariantControl=F==2
  Subsystem2 : Subsystem  VariantControl=F==3
  Out1 : Outport

== system PID_controler/pid5 ==
  In1 : Inport
  Subsystem : Subsystem  VariantControl=F==1
  Subsystem1 : Subsystem  VariantControl=F==2
  Subsystem2 : Subsystem  VariantControl=F==3
  Out1 : Outport

== system PID_controler/pid6 ==
  In1 : Inport
  Subsystem : Subsystem  VariantControl=F==1
  Subsystem1 : Subsystem  VariantControl=F==2
  Subsystem2 : Subsystem  VariantControl=F==3
  Out1 : Outport

== system PID_controler/pid7 ==
  In1 : Inport
  Subsystem : Subsystem  VariantControl=F==1
  Subsystem1 : Subsystem  VariantControl=F==2
  Subsystem2 : Subsystem  VariantControl=F==3
  Out1 : Outport

== system PID_controler/pid8 ==
  In1 : Inport
  Subsystem : Subsystem  VariantControl=F==1
  Subsystem1 : Subsystem  VariantControl=F==2
  Subsystem2 : Subsystem  VariantControl=F==3
  Out1 : Outport

== system PID_controler/pid9 ==
  In1 : Inport
  Subsystem : Subsystem  VariantControl=F==1
  Subsystem1 : Subsystem  VariantControl=F==2
  Subsystem2 : Subsystem  VariantControl=F==3
  Out1 : Outport

== system PID_controler/pid/Subsystem ==
  In1 : Inport
  Derivative : Derivative
  Gain : Gain  Gain=P
  Gain1 : Gain  Gain=I
  Gain2 : Gain  Gain=D
  Integrator : Integrator
  Sum : Sum  Inputs=+++
  Out1 : Outport
  wires:
  In1/1 -> Gain1/1, Gain2/1, Gain/1
  Derivative/1 -> Sum/3
  Gain/1 -> Sum/1
  Integrator/1 -> Sum/2
  Sum/1 -> Out1/1
  Gain2/1 -> Derivative/1
  Gain1/1 -> Integrator/1

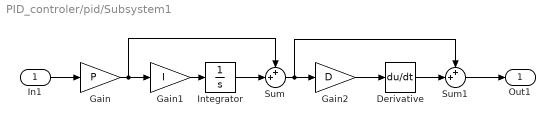
== system PID_controler/pid/Subsystem1 ==
  In1 : Inport
  Derivative : Derivative
  Gain : Gain  Gain=P
  Gain1 : Gain  Gain=I
  Gain2 : Gain  Gain=D
  Integrator : Integrator
  Sum : Sum  Inputs=++|
  Sum1 : Sum  Inputs=++|
  Out1 : Outport
  wires:
  Derivative/1 -> Sum1/2
  Sum1/1 -> Out1/1
  In1/1 -> Gain/1
  Gain1/1 -> Integrator/1
  Integrator/1 -> Sum/2
  Gain/1 -> Gain1/1, Sum/1
  Gain2/1 -> Derivative/1
  Sum/1 -> Gain2/1, Sum1/1

== system PID_controler/pid/Subsystem2 ==
  In1 : Inport
  Derivative : Derivative
  Gain : Gain  Gain=P
  Gain1 : Gain  Gain=I
  Gain2 : Gain  Gain=D
  Integrator : Integrator
  Sum : Sum  Inputs=+++
  Out1 : Outport
  wires:
  In1/1 -> Gain/1
  Sum/1 -> Out1/1
  Derivative/1 -> Sum/3
  Gain2/1 -> Derivative/1
  Integrator/1 -> Sum/2
  Gain1/1 -> Integrator/1
  Gain/1 -> Sum/1, Gain1/1, Gain2/1

== system PID_controler/pid1/Subsystem ==
  In1 : Inport
  Derivative : Derivative
  Gain : Gain  Gain=P
  Gain1 : Gain  Gain=I
  Gain2 : Gain  Gain=D
  Integrator : Integrator
  Sum : Sum  Inputs=+++
  Out1 : Outport
  wires:
  In1/1 -> Gain1/1, Gain2/1, Gain/1
  Derivative/1 -> Sum/3
  Gain/1 -> Sum/1
  Integrator/1 -> Sum/2
  Sum/1 -> Out1/1
  Gain2/1 -> Derivative/1
  Gain1/1 -> Integrator/1

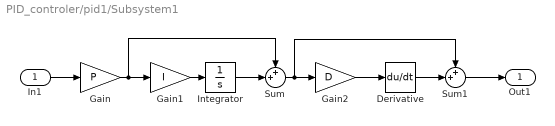
== system PID_controler/pid1/Subsystem1 ==
  In1 : Inport
  Derivative : Derivative
  Gain : Gain  Gain=P
  Gain1 : Gain  Gain=I
  Gain2 : Gain  Gain=D
  Integrator : Integrator
  Sum : Sum  Inputs=++|
  Sum1 : Sum  Inputs=++|
  Out1 : Outport
  wires:
  Derivative/1 -> Sum1/2
  Sum1/1 -> Out1/1
  In1/1 -> Gain/1
  Gain1/1 -> Integrator/1
  Integrator/1 -> Sum/2
  Gain/1 -> Gain1/1, Sum/1
  Gain2/1 -> Derivative/1
  Sum/1 -> Gain2/1, Sum1/1

== system PID_controler/pid1/Subsystem2 ==
  In1 : Inport
  Derivative : Derivative
  Gain : Gain  Gain=P
  Gain1 : Gain  Gain=I
  Gain2 : Gain  Gain=D
  Integrator : Integrator
  Sum : Sum  Inputs=+++
  Out1 : Outport
  wires:
  In1/1 -> Gain/1
  Sum/1 -> Out1/1
  Derivative/1 -> Sum/3
  Gain2/1 -> Derivative/1
  Integrator/1 -> Sum/2
  Gain1/1 -> Integrator/1
  Gain/1 -> Sum/1, Gain1/1, Gain2/1

== system PID_controler/pid10/Subsystem ==
  In1 : Inport
  Derivative : Derivative
  Gain : Gain  Gain=P
  Gain1 : Gain  Gain=I
  Gain2 : Gain  Gain=D
  Integrator : Integrator
  Sum : Sum  Inputs=+++
  Out1 : Outport
  wires:
  In1/1 -> Gain1/1, Gain2/1, Gain/1
  Derivative/1 -> Sum/3
  Gain/1 -> Sum/1
  Integrator/1 -> Sum/2
  Sum/1 -> Out1/1
  Gain2/1 -> Derivative/1
  Gain1/1 -> Integrator/1

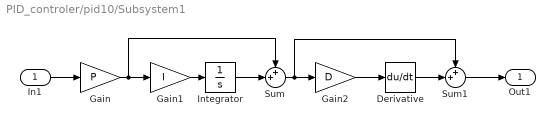
== system PID_controler/pid10/Subsystem1 ==
  In1 : Inport
  Derivative : Derivative
  Gain : Gain  Gain=P
  Gain1 : Gain  Gain=I
  Gain2 : Gain  Gain=D
  Integrator : Integrator
  Sum : Sum  Inputs=++|
  Sum1 : Sum  Inputs=++|
  Out1 : Outport
  wires:
  Derivative/1 -> Sum1/2
  Sum1/1 -> Out1/1
  In1/1 -> Gain/1
  Gain1/1 -> Integrator/1
  Integrator/1 -> Sum/2
  Gain/1 -> Gain1/1, Sum/1
  Gain2/1 -> Derivative/1
  Sum/1 -> Gain2/1, Sum1/1

== system PID_controler/pid10/Subsystem2 ==
  In1 : Inport
  Derivative : Derivative
  Gain : Gain  Gain=P
  Gain1 : Gain  Gain=I
  Gain2 : Gain  Gain=D
  Integrator : Integrator
  Sum : Sum  Inputs=+++
  Out1 : Outport
  wires:
  In1/1 -> Gain/1
  Sum/1 -> Out1/1
  Derivative/1 -> Sum/3
  Gain2/1 -> Derivative/1
  Integrator/1 -> Sum/2
  Gain1/1 -> Integrator/1
  Gain/1 -> Sum/1, Gain1/1, Gain2/1

== system PID_controler/pid11/Subsystem ==
  In1 : Inport
  Derivative : Derivative
  Gain : Gain  Gain=P
  Gain1 : Gain  Gain=I
  Gain2 : Gain  Gain=D
  Integrator : Integrator
  Sum : Sum  Inputs=+++
  Out1 : Outport
  wires:
  In1/1 -> Gain1/1, Gain2/1, Gain/1
  Derivative/1 -> Sum/3
  Gain/1 -> Sum/1
  Integrator/1 -> Sum/2
  Sum/1 -> Out1/1
  Gain2/1 -> Derivative/1
  Gain1/1 -> Integrator/1

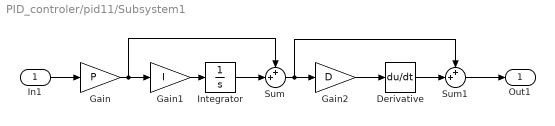
== system PID_controler/pid11/Subsystem1 ==
  In1 : Inport
  Derivative : Derivative
  Gain : Gain  Gain=P
  Gain1 : Gain  Gain=I
  Gain2 : Gain  Gain=D
  Integrator : Integrator
  Sum : Sum  Inputs=++|
  Sum1 : Sum  Inputs=++|
  Out1 : Outport
  wires:
  Derivative/1 -> Sum1/2
  Sum1/1 -> Out1/1
  In1/1 -> Gain/1
  Gain1/1 -> Integrator/1
  Integrator/1 -> Sum/2
  Gain/1 -> Gain1/1, Sum/1
  Gain2/1 -> Derivative/1
  Sum/1 -> Gain2/1, Sum1/1

== system PID_controler/pid11/Subsystem2 ==
  In1 : Inport
  Derivative : Derivative
  Gain : Gain  Gain=P
  Gain1 : Gain  Gain=I
  Gain2 : Gain  Gain=D
  Integrator : Integrator
  Sum : Sum  Inputs=+++
  Out1 : Outport
  wires:
  In1/1 -> Gain/1
  Sum/1 -> Out1/1
  Derivative/1 -> Sum/3
  Gain2/1 -> Derivative/1
  Integrator/1 -> Sum/2
  Gain1/1 -> Integrator/1
  Gain/1 -> Sum/1, Gain1/1, Gain2/1

== system PID_controler/pid12/Subsystem ==
  In1 : Inport
  Derivative : Derivative
  Gain : Gain  Gain=P
  Gain1 : Gain  Gain=I
  Gain2 : Gain  Gain=D
  Integrator : Integrator
  Sum : Sum  Inputs=+++
  Out1 : Outport
  wires:
  In1/1 -> Gain1/1, Gain2/1, Gain/1
  Derivative/1 -> Sum/3
  Gain/1 -> Sum/1
  Integrator/1 -> Sum/2
  Sum/1 -> Out1/1
  Gain2/1 -> Derivative/1
  Gain1/1 -> Integrator/1

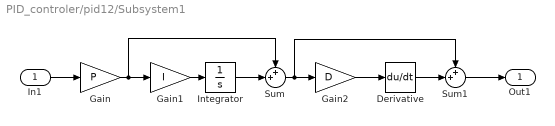
== system PID_controler/pid12/Subsystem1 ==
  In1 : Inport
  Derivative : Derivative
  Gain : Gain  Gain=P
  Gain1 : Gain  Gain=I
  Gain2 : Gain  Gain=D
  Integrator : Integrator
  Sum : Sum  Inputs=++|
  Sum1 : Sum  Inputs=++|
  Out1 : Outport
  wires:
  Derivative/1 -> Sum1/2
  Sum1/1 -> Out1/1
  In1/1 -> Gain/1
  Gain1/1 -> Integrator/1
  Integrator/1 -> Sum/2
  Gain/1 -> Gain1/1, Sum/1
  Gain2/1 -> Derivative/1
  Sum/1 -> Gain2/1, Sum1/1

== system PID_controler/pid12/Subsystem2 ==
  In1 : Inport
  Derivative : Derivative
  Gain : Gain  Gain=P
  Gain1 : Gain  Gain=I
  Gain2 : Gain  Gain=D
  Integrator : Integrator
  Sum : Sum  Inputs=+++
  Out1 : Outport
  wires:
  In1/1 -> Gain/1
  Sum/1 -> Out1/1
  Derivative/1 -> Sum/3
  Gain2/1 -> Derivative/1
  Integrator/1 -> Sum/2
  Gain1/1 -> Integrator/1
  Gain/1 -> Sum/1, Gain1/1, Gain2/1

== system PID_controler/pid13/Subsystem ==
  In1 : Inport
  Derivative : Derivative
  Gain : Gain  Gain=P
  Gain1 : Gain  Gain=I
  Gain2 : Gain  Gain=D
  Integrator : Integrator
  Sum : Sum  Inputs=+++
  Out1 : Outport
  wires:
  In1/1 -> Gain1/1, Gain2/1, Gain/1
  Derivative/1 -> Sum/3
  Gain/1 -> Sum/1
  Integrator/1 -> Sum/2
  Sum/1 -> Out1/1
  Gain2/1 -> Derivative/1
  Gain1/1 -> Integrator/1

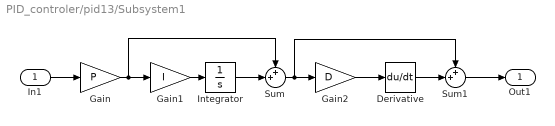
== system PID_controler/pid13/Subsystem1 ==
  In1 : Inport
  Derivative : Derivative
  Gain : Gain  Gain=P
  Gain1 : Gain  Gain=I
  Gain2 : Gain  Gain=D
  Integrator : Integrator
  Sum : Sum  Inputs=++|
  Sum1 : Sum  Inputs=++|
  Out1 : Outport
  wires:
  Derivative/1 -> Sum1/2
  Sum1/1 -> Out1/1
  In1/1 -> Gain/1
  Gain1/1 -> Integrator/1
  Integrator/1 -> Sum/2
  Gain/1 -> Gain1/1, Sum/1
  Gain2/1 -> Derivative/1
  Sum/1 -> Gain2/1, Sum1/1

== system PID_controler/pid13/Subsystem2 ==
  In1 : Inport
  Derivative : Derivative
  Gain : Gain  Gain=P
  Gain1 : Gain  Gain=I
  Gain2 : Gain  Gain=D
  Integrator : Integrator
  Sum : Sum  Inputs=+++
  Out1 : Outport
  wires:
  In1/1 -> Gain/1
  Sum/1 -> Out1/1
  Derivative/1 -> Sum/3
  Gain2/1 -> Derivative/1
  Integrator/1 -> Sum/2
  Gain1/1 -> Integrator/1
  Gain/1 -> Sum/1, Gain1/1, Gain2/1

== system PID_controler/pid14/Subsystem ==
  In1 : Inport
  Derivative : Derivative
  Gain : Gain  Gain=P
  Gain1 : Gain  Gain=I
  Gain2 : Gain  Gain=D
  Integrator : Integrator
  Sum : Sum  Inputs=+++
  Out1 : Outport
  wires:
  In1/1 -> Gain1/1, Gain2/1, Gain/1
  Derivative/1 -> Sum/3
  Gain/1 -> Sum/1
  Integrator/1 -> Sum/2
  Sum/1 -> Out1/1
  Gain2/1 -> Derivative/1
  Gain1/1 -> Integrator/1

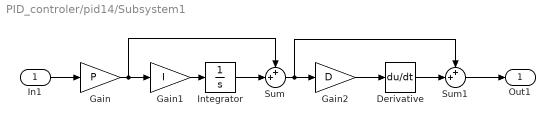
== system PID_controler/pid14/Subsystem1 ==
  In1 : Inport
  Derivative : Derivative
  Gain : Gain  Gain=P
  Gain1 : Gain  Gain=I
  Gain2 : Gain  Gain=D
  Integrator : Integrator
  Sum : Sum  Inputs=++|
  Sum1 : Sum  Inputs=++|
  Out1 : Outport
  wires:
  Derivative/1 -> Sum1/2
  Sum1/1 -> Out1/1
  In1/1 -> Gain/1
  Gain1/1 -> Integrator/1
  Integrator/1 -> Sum/2
  Gain/1 -> Gain1/1, Sum/1
  Gain2/1 -> Derivative/1
  Sum/1 -> Gain2/1, Sum1/1

== system PID_controler/pid14/Subsystem2 ==
  In1 : Inport
  Derivative : Derivative
  Gain : Gain  Gain=P
  Gain1 : Gain  Gain=I
  Gain2 : Gain  Gain=D
  Integrator : Integrator
  Sum : Sum  Inputs=+++
  Out1 : Outport
  wires:
  In1/1 -> Gain/1
  Sum/1 -> Out1/1
  Derivative/1 -> Sum/3
  Gain2/1 -> Derivative/1
  Integrator/1 -> Sum/2
  Gain1/1 -> Integrator/1
  Gain/1 -> Sum/1, Gain1/1, Gain2/1

== system PID_controler/pid15/Subsystem ==
  In1 : Inport
  Derivative : Derivative
  Gain : Gain  Gain=P
  Gain1 : Gain  Gain=I
  Gain2 : Gain  Gain=D
  Integrator : Integrator
  Sum : Sum  Inputs=+++
  Out1 : Outport
  wires:
  Gain1/1 -> Integrator/1
  Gain2/1 -> Derivative/1
  Sum/1 -> Out1/1
  Integrator/1 -> Sum/2
  Gain/1 -> Sum/1
  Derivative/1 -> Sum/3
  In1/1 -> Gain/1, Gain2/1, Gain1/1

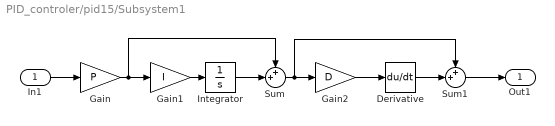
== system PID_controler/pid15/Subsystem1 ==
  In1 : Inport
  Derivative : Derivative
  Gain : Gain  Gain=P
  Gain1 : Gain  Gain=I
  Gain2 : Gain  Gain=D
  Integrator : Integrator
  Sum : Sum  Inputs=++|
  Sum1 : Sum  Inputs=++|
  Out1 : Outport
  wires:
  Sum/1 -> Sum1/1, Gain2/1
  Gain2/1 -> Derivative/1
  Gain/1 -> Sum/1, Gain1/1
  Integrator/1 -> Sum/2
  Gain1/1 -> Integrator/1
  In1/1 -> Gain/1
  Sum1/1 -> Out1/1
  Derivative/1 -> Sum1/2

== system PID_controler/pid15/Subsystem2 ==
  In1 : Inport
  Derivative : Derivative
  Gain : Gain  Gain=P
  Gain1 : Gain  Gain=I
  Gain2 : Gain  Gain=D
  Integrator : Integrator
  Sum : Sum  Inputs=+++
  Out1 : Outport
  wires:
  Gain/1 -> Gain2/1, Gain1/1, Sum/1
  Gain1/1 -> Integrator/1
  Integrator/1 -> Sum/2
  Gain2/1 -> Derivative/1
  Derivative/1 -> Sum/3
  Sum/1 -> Out1/1
  In1/1 -> Gain/1

== system PID_controler/pid16/Subsystem ==
  In1 : Inport
  Derivative : Derivative
  Gain : Gain  Gain=P
  Gain1 : Gain  Gain=I
  Gain2 : Gain  Gain=D
  Integrator : Integrator
  Sum : Sum  Inputs=+++
  Out1 : Outport
  wires:
  Gain1/1 -> Integrator/1
  Gain2/1 -> Derivative/1
  Sum/1 -> Out1/1
  Integrator/1 -> Sum/2
  Gain/1 -> Sum/1
  Derivative/1 -> Sum/3
  In1/1 -> Gain/1, Gain2/1, Gain1/1

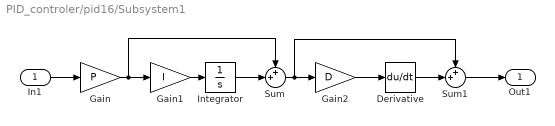
== system PID_controler/pid16/Subsystem1 ==
  In1 : Inport
  Derivative : Derivative
  Gain : Gain  Gain=P
  Gain1 : Gain  Gain=I
  Gain2 : Gain  Gain=D
  Integrator : Integrator
  Sum : Sum  Inputs=++|
  Sum1 : Sum  Inputs=++|
  Out1 : Outport
  wires:
  Sum/1 -> Sum1/1, Gain2/1
  Gain2/1 -> Derivative/1
  Gain/1 -> Sum/1, Gain1/1
  Integrator/1 -> Sum/2
  Gain1/1 -> Integrator/1
  In1/1 -> Gain/1
  Sum1/1 -> Out1/1
  Derivative/1 -> Sum1/2
